simulink model "SystemSim"  (R2015a)
settings: Solver=ode45  StartTime=0.0  StopTime=time  RelTol=1e-3
values from neighbouring files (symbols this model uses):
  C_a = poly(2)    [Estimation_script.m]
  D_d = poly(1)    [Estimation_script.m]
  g = 9.8    [Estimation_script.m]
  h = h_d = h_a    [Estimation_script.m]
  rho_a = (1/g*h)*avg_p_hdiff    [Estimation_script.m]
  rho_d = poly(3)/(g*h)    [Estimation_script.m]
settings Model: Creator=gardhi  LastModifiedBy=gardhi
settings SolverCC: MaxConsecutiveMinStep=2

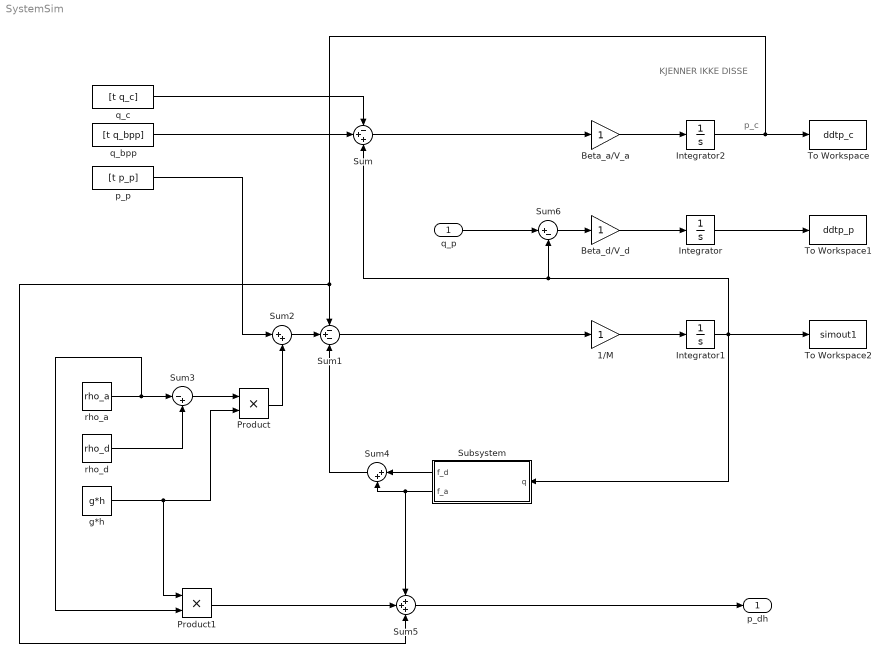
== system SystemSim ==
  note: KJENNER
      | IKKE
      | DISSE
  note: p_c
  "q_p " : Inport
  "1/M " : Gain
  "Beta_a/V_a " : Gain
  Beta_d/V_d : Gain
  Integrator : Integrator
  Integrator1 : Integrator
  Integrator2 : Integrator
  Product : Product
  Product1 : Product
  Subsystem : Subsystem
  Sum : Sum  Inputs=-++
  Sum1 : Sum  Inputs=-+-
  Sum2 : Sum  Inputs=|++
  Sum3 : Sum  Inputs=|-+
  Sum4 : Sum  Inputs=|++
  Sum5 : Sum  Inputs=+++
  Sum6 : Sum  Inputs=|+-
  To Workspace : ToWorkspace  VariableName=ddtp_c  SaveFormat=Timeseries  SampleTime=-1
  To Workspace1 : ToWorkspace  VariableName=ddtp_p  SaveFormat=Timeseries  SampleTime=-1
  To Workspace2 : ToWorkspace  VariableName=simout1  SaveFormat=Timeseries  SampleTime=-1
  g*h : Constant  Value=g*h
  p_p : FromWorkspace  VariableName=[t p_p]  SampleTime=0
  q_bpp : FromWorkspace  VariableName=[t q_bpp]  SampleTime=0
  q_c : FromWorkspace  VariableName=[t q_c]  SampleTime=0
  rho_a : Constant  Value=rho_a
  rho_d : Constant  Value=rho_d
  p_dh : Outport
  wires:
  Sum1/1 -> "1/M "/1
  q_bpp/1 -> Sum/2
  q_c/1 -> Sum/1
  Sum/1 -> "Beta_a/V_a "/1
  p_p/1 -> Sum2/1
  Sum2/1 -> Sum1/2
  rho_a/1 -> Product1/2, Sum3/1
  rho_d/1 -> Sum3/2
  Product/1 -> Sum2/2
  Sum3/1 -> Product/1
  g*h/1 -> Product1/1, Product/2
  Sum4/1 -> Sum1/3
  Product1/1 -> Sum5/2
  Sum5/1 -> p_dh/1
  "q_p "/1 -> Sum6/1
  Sum6/1 -> Beta_d/V_d/1
  Subsystem/1(f_d) -> Sum4/1
  Subsystem/2(f_a) -> Sum5/1, Sum4/2
  "Beta_a/V_a "/1 -> Integrator2/1
  Beta_d/V_d/1 -> Integrator/1
  "1/M "/1 -> Integrator1/1
  Integrator2/1 -> Sum5/3, Sum1/1, To Workspace/1
  Integrator/1 -> To Workspace1/1
  Integrator1/1 -> Subsystem/1(q), To Workspace2/1, Sum/3, Sum6/2

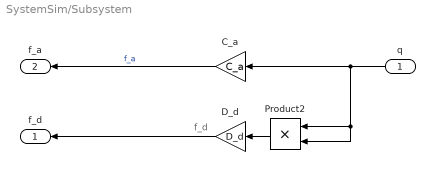
== system SystemSim/Subsystem ==
  note: f_d
  q : Inport
  C_a : Gain  Gain=C_a
  D_d : Gain  Gain=D_d
  Product2 : Product
  f_d : Outport
  f_a : Outport  Port=2
  wires:
  D_d/1 -> f_d/1
  C_a/1 -> f_a/1  "f_a"
  Product2/1 -> D_d/1
  q/1 -> Product2/1, Product2/2, C_a/1
